simulink model "HistoryJunctionAnalyzerTest"  (Simulink 6.3)
settings: Solver=ode45  StartTime=0.0  StopTime=10.0  RelTol=1e-3
settings Model: LastModifiedBy=deissenb

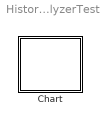
== system HistoryJunctionAnalyzerTest ==
  Chart : Stateflow chart

== stateflow chart Chart ==
  state ?
  state ?
  ? -> (history)
  (history) -> ?
